simulink model "zadaca2Simulink"  (R2018a)
settings: Solver=VariableStepAuto  StartTime=0.0  StopTime=10.0  RelTol=1e-3
settings Model: Creator=User  LastModifiedBy=User

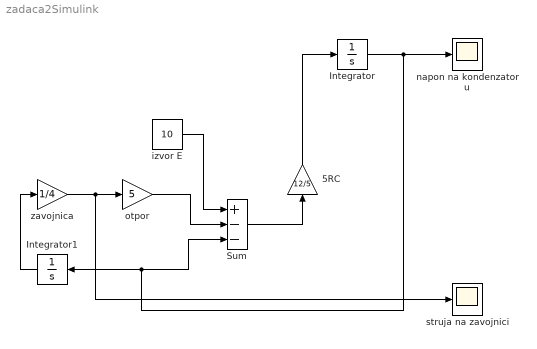
== system zadaca2Simulink ==
  5RC : Gain  Gain=12/5
  Integrator : Integrator
  Integrator1 : Integrator
  Sum : Sum  Inputs=+--
  izvor E : Constant  Value=10
  "napon na kondenzatoru " : Scope
  otpor : Gain  Gain=5
  struja na zavojnici : Scope
  "zavojnica " : Gain  Gain=1/4
  wires:
  5RC/1 -> Integrator/1
  Sum/1 -> 5RC/1
  "zavojnica "/1 -> struja na zavojnici/1, otpor/1
  Integrator1/1 -> "zavojnica "/1
  Integrator/1 -> "napon na kondenzatoru "/1, Sum/3, Integrator1/1
  otpor/1 -> Sum/2
  izvor E/1 -> Sum/1
